simulink model "values_separater"  (R2016b)
settings: Solver=FixedStepAuto  StartTime=0.0  StopTime=inf  FixedStep=.01  RelTol=1e-3  SampleTimeConstraint=STIndependent
libraries: robotlib x11
settings Model: Creator=mph  LastModifiedBy=mph

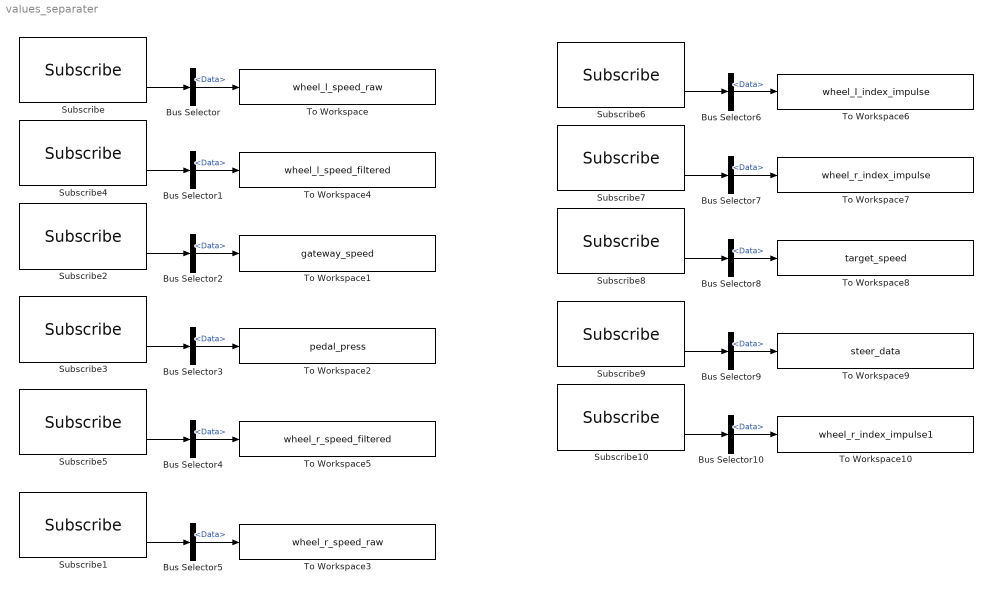
== system values_separater ==
  Bus Selector{,1..10} (11 alike) : BusSelector  OutputSignals=Data
  Subscribe : robotlib/Subscribe  SourceLibraryInfo=This block requires Robotics System Toolbox  topicSource=Select from ROS network  topic=/sep/wheel_l/speed_unfiltered  messageType=std_msgs/Float64  sampleTime=-1  messageQueueLength=1
  Subscribe1 : robotlib/Subscribe  SourceLibraryInfo=This block requires Robotics System Toolbox  topicSource=Select from ROS network  topic=/sep/wheel_r/speed_unfiltered  messageType=std_msgs/Float64  sampleTime=-1  messageQueueLength=1
  Subscribe10 : robotlib/Subscribe  SourceLibraryInfo=This block requires Robotics System Toolbox  topicSource=Select from ROS network  topic=/brake_in  messageType=std_msgs/Int64  sampleTime=-1  messageQueueLength=1
  Subscribe2 : robotlib/Subscribe  SourceLibraryInfo=This block requires Robotics System Toolbox  topicSource=Select from ROS network  topic=/speed  messageType=std_msgs/Float64  sampleTime=-1  messageQueueLength=1
  Subscribe3 : robotlib/Subscribe  SourceLibraryInfo=This block requires Robotics System Toolbox  topicSource=Select from ROS network  topic=/accl_in  messageType=std_msgs/Int64  sampleTime=-1  messageQueueLength=1
  Subscribe4 : robotlib/Subscribe  SourceLibraryInfo=This block requires Robotics System Toolbox  topicSource=Select from ROS network  topic=/sep/wheel_l/speed  messageType=std_msgs/Float64  sampleTime=-1  messageQueueLength=1
  Subscribe5 : robotlib/Subscribe  SourceLibraryInfo=This block requires Robotics System Toolbox  topicSource=Select from ROS network  topic=/sep/wheel_r/speed  messageType=std_msgs/Float64  sampleTime=-1  messageQueueLength=1
  Subscribe6 : robotlib/Subscribe  SourceLibraryInfo=This block requires Robotics System Toolbox  topicSource=Select from ROS network  topic=/sep/wheel_l/index_count_zero  messageType=std_msgs/Float64  sampleTime=-1  messageQueueLength=1
  Subscribe7 : robotlib/Subscribe  SourceLibraryInfo=This block requires Robotics System Toolbox  topicSource=Select from ROS network  topic=/sep/wheel_r/index_count_zero  messageType=std_msgs/Float64  sampleTime=-1  messageQueueLength=1
  Subscribe8 : robotlib/Subscribe  SourceLibraryInfo=This block requires Robotics System Toolbox  topicSource=Select from ROS network  topic=/can/control_velocity_2  messageType=std_msgs/Int64  sampleTime=-1  messageQueueLength=1
  Subscribe9 : robotlib/Subscribe  SourceLibraryInfo=This block requires Robotics System Toolbox  topicSource=Select from ROS network  topic=/steer_in  messageType=std_msgs/Int64  sampleTime=-1  messageQueueLength=1
  To Workspace : ToWorkspace  VariableName=wheel_l_speed_raw  SampleTime=-1
  To Workspace1 : ToWorkspace  VariableName=gateway_speed  SampleTime=-1
  To Workspace10 : ToWorkspace  VariableName=wheel_r_index_impulse1  SampleTime=-1
  To Workspace2 : ToWorkspace  VariableName=pedal_press  SampleTime=-1
  To Workspace3 : ToWorkspace  VariableName=wheel_r_speed_raw  SampleTime=-1
  To Workspace4 : ToWorkspace  VariableName=wheel_l_speed_filtered  SampleTime=-1
  To Workspace5 : ToWorkspace  VariableName=wheel_r_speed_filtered  SampleTime=-1
  To Workspace6 : ToWorkspace  VariableName=wheel_l_index_impulse  SampleTime=-1
  To Workspace7 : ToWorkspace  VariableName=wheel_r_index_impulse  SampleTime=-1
  To Workspace8 : ToWorkspace  VariableName=target_speed  SampleTime=-1
  To Workspace9 : ToWorkspace  VariableName=steer_data  SampleTime=-1
  wires:
  Subscribe/2 -> Bus Selector/1
  Bus Selector/1 -> To Workspace/1  "<Data>"
  Subscribe4/2 -> Bus Selector1/1
  Bus Selector1/1 -> To Workspace4/1  "<Data>"
  Subscribe2/2 -> Bus Selector2/1
  Bus Selector2/1 -> To Workspace1/1  "<Data>"
  Subscribe3/2 -> Bus Selector3/1
  Bus Selector3/1 -> To Workspace2/1  "<Data>"
  Subscribe5/2 -> Bus Selector4/1
  Bus Selector4/1 -> To Workspace5/1  "<Data>"
  Subscribe1/2 -> Bus Selector5/1
  Bus Selector5/1 -> To Workspace3/1  "<Data>"
  Subscribe6/2 -> Bus Selector6/1
  Bus Selector6/1 -> To Workspace6/1  "<Data>"
  Subscribe7/2 -> Bus Selector7/1
  Bus Selector7/1 -> To Workspace7/1  "<Data>"
  Subscribe8/2 -> Bus Selector8/1
  Bus Selector8/1 -> To Workspace8/1  "<Data>"
  Subscribe9/2 -> Bus Selector9/1
  Bus Selector9/1 -> To Workspace9/1  "<Data>"
  Subscribe10/2 -> Bus Selector10/1
  Bus Selector10/1 -> To Workspace10/1  "<Data>"
